simulink model "csu_taf_thruster_arm_fire_hrn"  (R2014b)
settings: Solver=FixedStepDiscrete  StartTime=t0  StopTime=tFinal  FixedStep=sim_dt  RelTol=1e-3
libraries: util_info_lib x1, util_common_lib x1, csu_taf_thruster_arm_fire_lib x1
settings Model: Creator=escrane  LastModifiedBy=mstewart
settings DebuggingCC: UnderspecifiedInitializationDetection=Classic  MergeDetectMultiDrivingBlocksExec=none  InheritedTsInSrcMsg=none

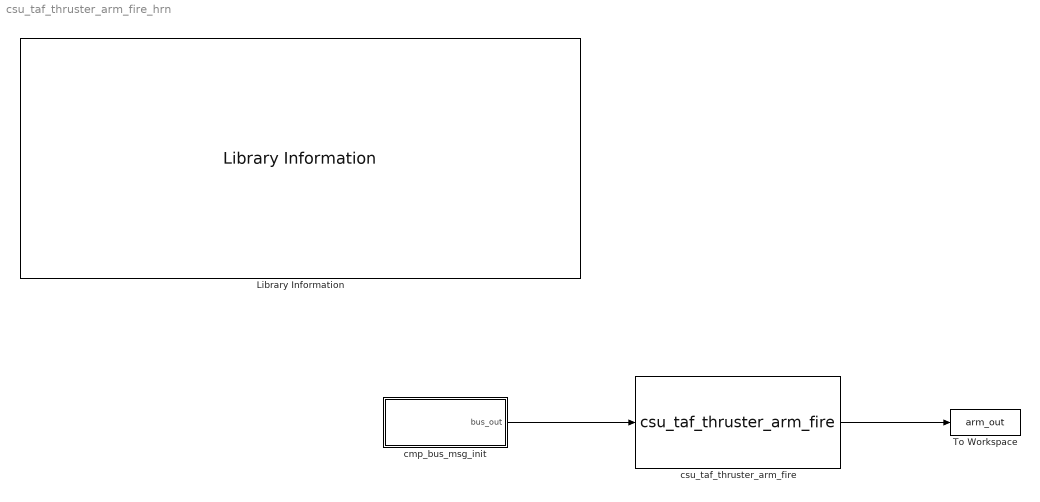
== system csu_taf_thruster_arm_fire_hrn ==
  Library Information : util_info_lib/Library Information  owner='escrane'
  To Workspace : ToWorkspace  VariableName=arm_out  SaveFormat=Timeseries  SampleTime=-1
  cmp_bus_msg_init : Subsystem
  csu_taf_thruster_arm_fire : csu_taf_thruster_arm_fire_lib/csu_taf_thruster_arm_fire
  wires:
  csu_taf_thruster_arm_fire/1 -> To Workspace/1
  cmp_bus_msg_init/1(bus_out) -> csu_taf_thruster_arm_fire/1

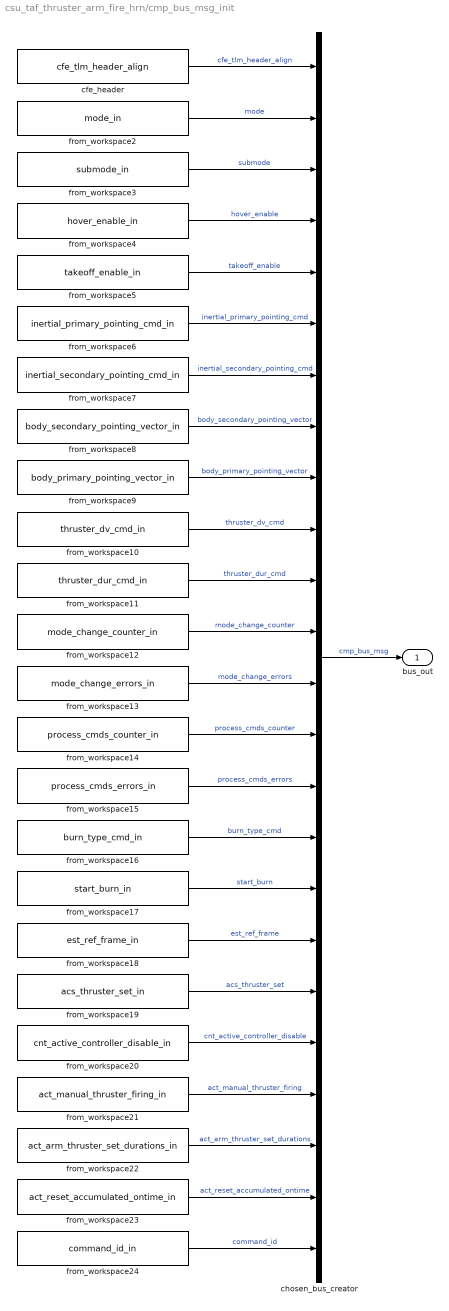
== system csu_taf_thruster_arm_fire_hrn/cmp_bus_msg_init ==
  cfe_header : util_common_lib/cfe_tlm_header_align
  chosen_bus_creator : BusCreator  Inputs=24  OutDataTypeStr=Bus: cmp_bus_msg  NonVirtualBus=on
  from_workspace10 : FromWorkspace  VariableName=thruster_dv_cmd_in
  from_workspace11 : FromWorkspace  VariableName=thruster_dur_cmd_in
  from_workspace12 : FromWorkspace  VariableName=mode_change_counter_in
  from_workspace13 : FromWorkspace  VariableName=mode_change_errors_in
  from_workspace14 : FromWorkspace  VariableName=process_cmds_counter_in
  from_workspace15 : FromWorkspace  VariableName=process_cmds_errors_in
  from_workspace16 : FromWorkspace  VariableName=burn_type_cmd_in
  from_workspace17 : FromWorkspace  VariableName=start_burn_in
  from_workspace18 : FromWorkspace  VariableName=est_ref_frame_in
  from_workspace19 : FromWorkspace  VariableName=acs_thruster_set_in
  from_workspace2 : FromWorkspace  VariableName=mode_in
  from_workspace20 : FromWorkspace  VariableName=cnt_active_controller_disable_in
  from_workspace21 : FromWorkspace  VariableName=act_manual_thruster_firing_in
  from_workspace22 : FromWorkspace  VariableName=act_arm_thruster_set_durations_in
  from_workspace23 : FromWorkspace  VariableName=act_reset_accumulated_ontime_in
  from_workspace24 : FromWorkspace  VariableName=command_id_in
  from_workspace3 : FromWorkspace  VariableName=submode_in
  from_workspace4 : FromWorkspace  VariableName=hover_enable_in
  from_workspace5 : FromWorkspace  VariableName=takeoff_enable_in
  from_workspace6 : FromWorkspace  VariableName=inertial_primary_pointing_cmd_in
  from_workspace7 : FromWorkspace  VariableName=inertial_secondary_pointing_cmd_in
  from_workspace8 : FromWorkspace  VariableName=body_secondary_pointing_vector_in
  from_workspace9 : FromWorkspace  VariableName=body_primary_pointing_vector_in
  bus_out : Outport
  wires:
  from_workspace24/1 -> chosen_bus_creator/24  "command_id"
  from_workspace23/1 -> chosen_bus_creator/23  "act_reset_accumulated_ontime"
  from_workspace22/1 -> chosen_bus_creator/22  "act_arm_thruster_set_durations"
  from_workspace21/1 -> chosen_bus_creator/21  "act_manual_thruster_firing"
  from_workspace20/1 -> chosen_bus_creator/20  "cnt_active_controller_disable"
  from_workspace19/1 -> chosen_bus_creator/19  "acs_thruster_set"
  from_workspace18/1 -> chosen_bus_creator/18  "est_ref_frame"
  from_workspace17/1 -> chosen_bus_creator/17  "start_burn"
  from_workspace16/1 -> chosen_bus_creator/16  "burn_type_cmd"
  from_workspace15/1 -> chosen_bus_creator/15  "process_cmds_errors"
  from_workspace14/1 -> chosen_bus_creator/14  "process_cmds_counter"
  from_workspace13/1 -> chosen_bus_creator/13  "mode_change_errors"
  from_workspace12/1 -> chosen_bus_creator/12  "mode_change_counter"
  from_workspace11/1 -> chosen_bus_creator/11  "thruster_dur_cmd"
  from_workspace10/1 -> chosen_bus_creator/10  "thruster_dv_cmd"
  from_workspace9/1 -> chosen_bus_creator/9  "body_primary_pointing_vector"
  from_workspace8/1 -> chosen_bus_creator/8  "body_secondary_pointing_vector"
  from_workspace7/1 -> chosen_bus_creator/7  "inertial_secondary_pointing_cmd"
  from_workspace6/1 -> chosen_bus_creator/6  "inertial_primary_pointing_cmd"
  from_workspace5/1 -> chosen_bus_creator/5  "takeoff_enable"
  from_workspace4/1 -> chosen_bus_creator/4  "hover_enable"
  from_workspace3/1 -> chosen_bus_creator/3  "submode"
  from_workspace2/1 -> chosen_bus_creator/2  "mode"
  cfe_header/1 -> chosen_bus_creator/1  "cfe_tlm_header_align"
  chosen_bus_creator/1 -> bus_out/1  "cmp_bus_msg"
